simulink model "uavR_R_beta"  (R2024a)
settings: Solver=ode45  StartTime=0.0  StopTime=20  RelTol=1e-3  EnableMultiTasking=on
values from neighbouring files (symbols this model uses):
  alate = [-0.664377411201 -330.163387746 53.2835973356 0 0 24.9999999996 0.0408233020992 -32.3114507249 0.453859073573 1 0 0 ... (36 elements, 6x6)]    [data.mat]    (also in uavck_0.3ma.mat = [-0.227087280821 0 0 -76.755540132 38.6889917334 100.9303781)
  blate = [0  0; -3.47475022598  0.138298516457; 0.0522368492882  -0.439264414469; 0  0; 0  0; 0  0]    [data.mat]    (also in uavck_0.3ma.mat = [0.000494526671357  0.00154149546586; 0  0; 0  0; -4.1487737)
  clate = [57.2957795131 0 0 0 0 0 0 57.2957795131 0 0 0 0 ... (36 elements, 6x6)]    [data.mat]    (also in uavck_0.3ma.mat = [57.2957804904 0 0 0 0 0 0 57.2957804904 0 0 0 0 ... (36 ele)
  dlate = [0  0; 0  0; 0  0; 0  0; 0  0; 0  0]    [data.mat]    (also in uavck_0.3ma.mat)
settings Model: Creator=Administrator  LastModifiedBy=rzxha
settings SolverCC: AlgebraicLoopSolver=TrustRegion
settings DataIOCC: SaveFormat=Array  SignalLoggingSaveFormat=ModelDataLogs  ReturnWorkspaceOutputs=off  SignalLoggingName=sigsOut
settings OptimizationCC: BooleanDataType=off  ExpressionDepthLimit=2147483647  InitFltsAndDblsToZero=on  LifeSpan=inf
settings DebuggingCC: SaveWithParameterizedLinksMsg=none  UnderspecifiedInitializationDetection=Classic  MergeDetectMultiDrivingBlocksExec=none  SignalResolutionControl=TryResolveAllWithWarning  MultiTaskDSMMsg=warning  MultiTaskCondExecSysMsg=none  FcnCallInpInsideContextMsg=warning  UnconnectedInputMsg=warning  UnconnectedOutputMsg=warning  UnconnectedLineMsg=warning  StateNameClashWarn=warning  SFUnexpectedBacktrackingDiag=warning  SFNoUnconditionalDefaultTransitionDiag=warning  ArithmeticOperatorsInVariantConditions=warning
settings HardwareCC: ProdBitPerPointer=32  ProdBitPerSizeT=32  ProdBitPerPtrDiffT=32  ProdLargestAtomicFloat=None  ProdIntDivRoundTo=Undefined  ProdEndianess=Unspecified  ProdWordSize=32  ProdHWDeviceType=32-bit Generic  TargetUnknown=on
settings ModelReferenceCC: EnableRefExpFcnMdlSchedulingChecks=on  PropagateSignalLabelsOutOfModel=off
settings SFSimCC: SimUseLocalCustomCode=off  CustomCodeUndefinedFunction=UseInterfaceOnly
settings RTWCC: RTWUseLocalCustomCode=off  GPUComputeCapability=3.5
settings CodeAppCC: StateflowObjectComments=on
settings GRTTargetCC: TargetFcnLib=ansi_tfl_tmw.mat  TargetLangStandard=C89/C90 (ANSI)  CombineOutputUpdateFcns=off  GRTInterface=on
settings ConfigComp: CovMetricSettings=dw  CovSaveCumulativeToWorkspaceVar=on  CovSaveSingleToWorkspaceVar=on  CovExternalEMLEnable=off

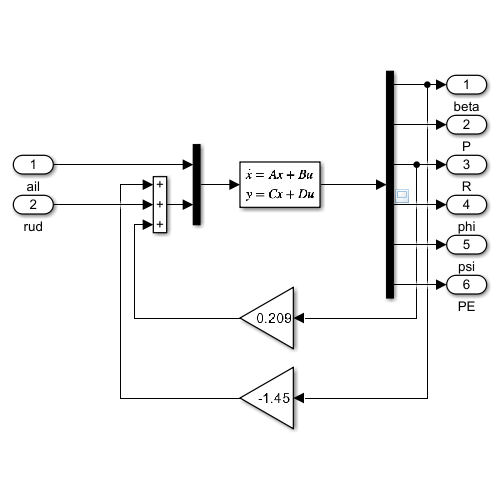
[thumbnail: Simulink's stored preview of the top-level diagram]
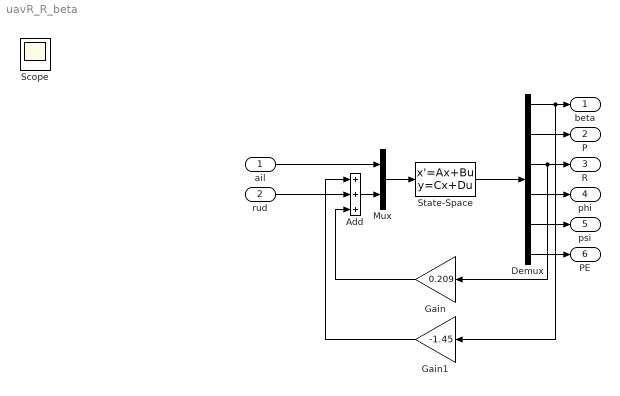
== system uavR_R_beta ==
  ail : Inport
  rud : Inport  Port=2
  Add : Sum  Inputs=+++
  Demux : Demux  Outputs=6
  Gain : Gain  Gain=0.209
  Gain1 : Gain  Gain=-1.45
  Mux : Mux  Inputs=2
  State-Space : StateSpace  A=alate  B=blate  C=clate  D=dlate  InitialCondition=0
  beta : Outport  VectorParamsAs1DForOutWhenUnconnected=off
  P : Outport  Port=2  VectorParamsAs1DForOutWhenUnconnected=off
  R : Outport  Port=3  VectorParamsAs1DForOutWhenUnconnected=off
  phi : Outport  Port=4  VectorParamsAs1DForOutWhenUnconnected=off
  psi : Outport  Port=5  VectorParamsAs1DForOutWhenUnconnected=off
  PE : Outport  Port=6  VectorParamsAs1DForOutWhenUnconnected=off
  Scope : Scope
  wires:
  Demux/1 -> Gain1/1, beta/1
  Demux/3 -> R/1, Gain/1
  Demux/4 -> phi/1
  Demux/5 -> psi/1
  Demux/2 -> P/1
  State-Space/1 -> Demux/1
  Mux/1 -> State-Space/1
  Demux/6 -> PE/1
  Add/1 -> Mux/2
  Gain1/1 -> Add/1
  Gain/1 -> Add/3
  ail/1 -> Mux/1
  rud/1 -> Add/2
